simulink model "GDFLIB_FilterIIR1_BAM_FLT"  (Simulink 8.3)
settings: Solver=ode45  StartTime=0.0  StopTime=10.0  RelTol=1e-3
undefined symbols (not defined in the file): fltA1, fltB0, fltB1
settings Model: Creator=B17364  LastModifiedBy=B17364
settings OptimizationCC: ExpressionDepthLimit=2147483647
settings DebuggingCC: FcnCallInpInsideContextMsg=UseLocalSettings  StrictBusMsg=Warning

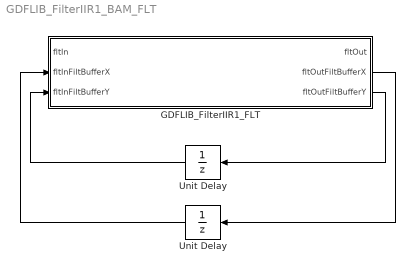
== system GDFLIB_FilterIIR1_BAM_FLT ==
  GDFLIB_FilterIIR1_FLT : Subsystem  mask(GDFLIB_FilterIIR1){fltB0=fltB0, fltB1=fltB1, fltA1=fltA1}
      mask help: Bit accurate model of first order IIR filter. All parameters as well as input and output are in single precision floating data format.
      mask init:
      | pos = get_param(gcb, 'Position');width = pos(3) - pos(1); height = pos(4) - pos(2);tX=width/2;tY=height*0.9;
      mask Display: color('black');port_label('input',1,'fltIn');port_label('input',2,'fltInFiltBufferX');port_label('input',3,'fltInFiltBufferY');port_label('output',1,'fltOut');port_label('output',2,'fltOutFiltBufferX');port_label('output',3,'fltOutFiltBufferY');color('black');disp('GDFLIB_FilterIIR1_FLT');color('blue');text(tX,tY, 'BAM', 'horizontalAlignment', 'center');
  Unit Delay : UnitDelay  SampleTime=-1
  "Unit Delay " : UnitDelay  SampleTime=-1
  wires:
  GDFLIB_FilterIIR1_FLT/2(fltOutFiltBufferX) -> "Unit Delay "/1
  "Unit Delay "/1 -> GDFLIB_FilterIIR1_FLT/2(fltInFiltBufferX)
  GDFLIB_FilterIIR1_FLT/3(fltOutFiltBufferY) -> Unit Delay/1
  Unit Delay/1 -> GDFLIB_FilterIIR1_FLT/3(fltInFiltBufferY)

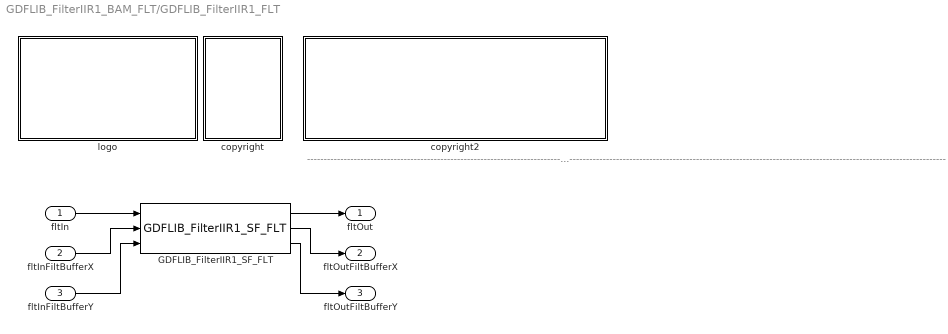
== system GDFLIB_FilterIIR1_BAM_FLT/GDFLIB_FilterIIR1_FLT ==
  note: ---------------------------------------------------------------------------------------------------------------------------------------------------------------------------------------------------
  fltIn : Inport
  fltInFiltBufferX : Inport  Port=2
  fltInFiltBufferY : Inport  Port=3
  GDFLIB_FilterIIR1_SF_FLT : S-Function  FunctionName=GDFLIB_FilterIIR1_SF_FLT  Parameters=fltB0,fltB1,fltA1  EnableBusSupport=off
  copyright : Subsystem
      mask Display:
      | text(10,90,'FILE:');text(10,75,'DESRIPTION:')
      | text(10,60,'COPYRIGHT:')
      | text(10,45,'VERSION:')
      | text(10,30,'DATE:')
      | text(10,15,'AUTHOR:')
  copyright2 : Subsystem
      mask Display:
      | text(10,90,'GDFLIB_FilterIIR1_BAM_FLT.mdl');text(10,75,'Direct form I first order IIR filter.');text(10,60,'Freescale')
      | text(10,45,'0.1');text(10,30,'08-Apr-2014');text(10,15,'');
  logo : Subsystem
      mask Display: image(imread('logo.jpg'))
  fltOut : Outport
  fltOutFiltBufferX : Outport  Port=2
  fltOutFiltBufferY : Outport  Port=3
  wires:
  fltIn/1 -> GDFLIB_FilterIIR1_SF_FLT/1
  GDFLIB_FilterIIR1_SF_FLT/1 -> fltOut/1
  GDFLIB_FilterIIR1_SF_FLT/2 -> fltOutFiltBufferX/1
  GDFLIB_FilterIIR1_SF_FLT/3 -> fltOutFiltBufferY/1
  fltInFiltBufferX/1 -> GDFLIB_FilterIIR1_SF_FLT/2
  fltInFiltBufferY/1 -> GDFLIB_FilterIIR1_SF_FLT/3

== system GDFLIB_FilterIIR1_BAM_FLT/GDFLIB_FilterIIR1_FLT/copyright ==

== system GDFLIB_FilterIIR1_BAM_FLT/GDFLIB_FilterIIR1_FLT/copyright2 ==

== system GDFLIB_FilterIIR1_BAM_FLT/GDFLIB_FilterIIR1_FLT/logo ==
